simulink model "SimProgetto"  (R2020a)
settings: Solver=VariableStepAuto  StartTime=0.0  StopTime=10  RelTol=1e-3
values from neighbouring files (symbols this model uses):
  Ae = [ 0                , 1 ... (first row only)    [Progetto1c.m]
  amplitude_n = 0.03    [Progetto1c.m]
  Be = [  0 ... (first row only)    [Progetto1c.m]
  Ce = [1,0]    [Progetto1c.m]
  den_g = d_g{1}    [Progetto1c.m]
  den_r = d_r{1}    [Progetto1c.m]
  num_g = n_g{1}    [Progetto1c.m]
  num_r = n_r{1}    [Progetto1c.m]
  omega_n = 2e04    (= 20000)    [Progetto1c.m]
  u_e = -1/2*sin(x1_e) * Fv    [Progetto1c.m]
  W = i    [Progetto1c.m]
  x0 = [theta_e;0]    [Progetto1c.m]
  y_e = x1_e    (= -0.523598775598)    [Progetto1c.m]
settings Model: Creator=De Luca  LastModifiedBy=De Luca

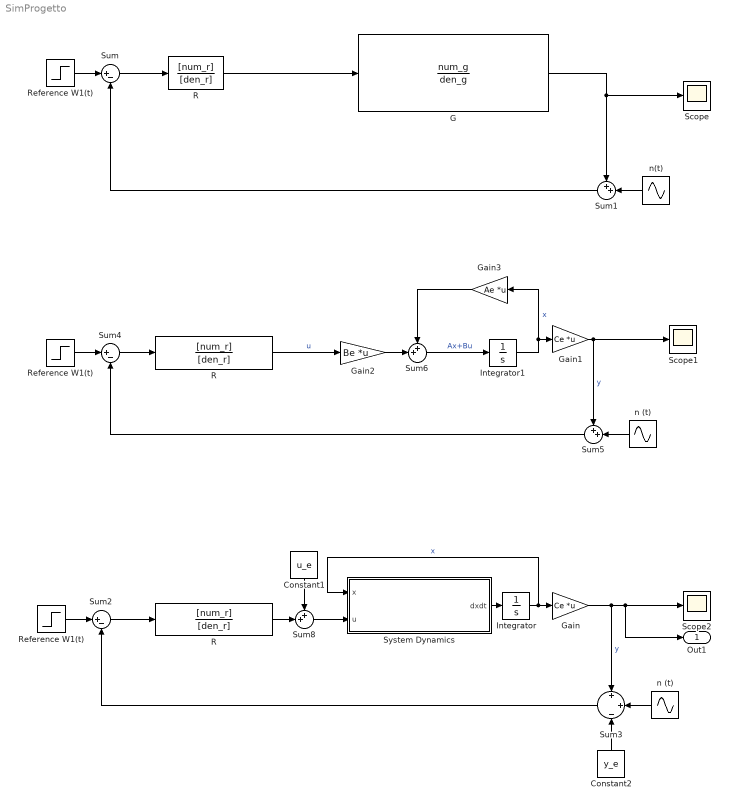
== system SimProgetto ==
  Constant1 : Constant  Value=u_e
  Constant2 : Constant  Value=y_e
  G : TransferFcn  Numerator=num_g  Denominator=den_g
  Gain : Gain  Gain=Ce  Multiplication=Matrix(K*u)
  Gain1 : Gain  Gain=Ce  Multiplication=Matrix(K*u)
  Gain2 : Gain  Gain=Be  Multiplication=Matrix(K*u)
  Gain3 : Gain  Gain=Ae  Multiplication=Matrix(K*u)
  Integrator : Integrator  InitialCondition=x0
  Integrator1 : Integrator  InitialCondition=x0
  R : TransferFcn  Numerator=[num_r]  Denominator=[den_r]
  "R " : TransferFcn  Numerator=[num_r]  Denominator=[den_r]
  "R " : TransferFcn  Numerator=[num_r]  Denominator=[den_r]
  Reference W1(t) : Step  Time=0  After=W  SampleTime=0
  "Reference W1(t) " : Step  Time=0  After=W  SampleTime=0
  "Reference W1(t) " : Step  Time=0  After=W  SampleTime=0
  Scope : Scope
  Scope1 : Scope
  Scope2 : Scope
  Sum : Sum  Inputs=|+-
  Sum{1,5..6,8} (4 alike) : Sum  Inputs=++|
  Sum2 : Sum  Inputs=|+-
  Sum3 : Sum  Inputs=+|+|-
  Sum4 : Sum  Inputs=|+-
  System Dynamics : MATLAB Function  TreatAsAtomicUnit=on
  n (t) : Sin  Amplitude=amplitude_n  Frequency=omega_n  SampleTime=0
  "n (t) " : Sin  Amplitude=amplitude_n  Frequency=omega_n  SampleTime=0
  n(t) : Sin  Amplitude=amplitude_n  Frequency=omega_n  SampleTime=0
  Out1 : Outport
  wires:
  G/1 -> Scope/1, Sum1/1
  Sum/1 -> R/1
  n(t)/1 -> Sum1/2
  R/1 -> G/1
  Sum1/1 -> Sum/2
  Reference W1(t)/1 -> Sum/1
  Sum5/1 -> Sum4/2
  Gain2/1 -> Sum6/2
  Gain3/1 -> Sum6/1
  "R "/1 -> Gain2/1  "u"
  "Reference W1(t) "/1 -> Sum4/1
  Integrator1/1 -> Gain1/1, Gain3/1  "x"
  Sum6/1 -> Integrator1/1  "Ax+Bu"
  "n (t) "/1 -> Sum5/2
  Gain1/1 -> Sum5/1, Scope1/1  "y"
  Sum4/1 -> "R "/1
  Sum3/1 -> Sum2/2
  n (t)/1 -> Sum3/2
  Sum2/1 -> "R "/1
  Gain/1 -> Out1/1, Scope2/1, Sum3/1  "y"
  "Reference W1(t) "/1 -> Sum2/1
  Integrator/1 -> System Dynamics/1(x), Gain/1  "x"
  System Dynamics/1(dxdt) -> Integrator/1
  "R "/1 -> Sum8/2
  Constant1/1 -> Sum8/1
  Sum8/1 -> System Dynamics/2(u)
  Constant2/1 -> Sum3/3

== matlab function SimProgetto/System Dynamics ==
  data: x input; u input; dxdt output
function dxdt = systemDynamics(x,u)
Fv = -13 ;      % forza del vento laterale
Id = 0.3 ;      % momento di inerzia del drone rispetto all'asse di rotazione
beta = 0.3;     % coefficiente di atrito dinamico
a = 0.25;       % distanza fra baricentro e applicazione della forza dei motori

dx1dt= x(2);
dx2dt= a/2*sin(x(1))*Fv/Id -beta/Id*x(2) + a/Id * u;
%dxdt = [dx1dt; dx2dt; dx3dt;...;dxndt];
dxdt = [dx1dt; dx2dt;];
